simulink model "Ex21"  (R2019b)
settings: Solver=VariableStepAuto  StartTime=0.0  StopTime=10  RelTol=1e-3
values from neighbouring files (symbols this model uses):
  f = 3    [Ex_20.m]    (also in Ex_21.m; Ex_8.m = [0.1 1 1.6 3 16]*1e3; Ex_9.m = 10.^(1 : 0.01 : 5))
  G = 9.8    [Ex_20.m]    (also in Ex_21.m)
  J = 0.4    [Ex_21.m]    (also in Ex_22.m = 1; Ex_23.m = 1.1; Ex_29.m = 1.1; Untitled2.m = 1)
  K = 1    [Ex_10.m]    (also in Ex_21.m; Ex_22.m; Ex_24.m = 1 / qsi^2; Ex_31.m = 4.26)
  M1 = 400    [Ex_20.m]    (also in Ex_21.m = 0.5; Untitled2.m = 1)
  M2 = 20    [Ex_20.m]    (also in Ex_21.m = 1; Untitled2.m = 1)
  R = 0.2    [Ex_21.m]    (also in Ex_22.m; Ex_23.m = 1.3; Ex_27.m = 2*qsi * sqrt(L/C); Ex_29.m = 1.3)
settings Model: Creator=andre  LastModifiedBy=andre

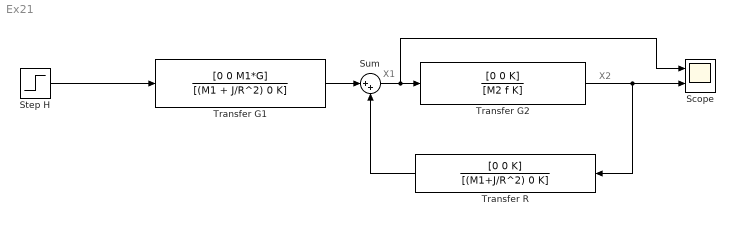
== system Ex21 ==
  note: X1
  note: X2
  Scope : Scope  NumInputPorts=2
  Step H : Step  Time=0  SampleTime=0
  Sum : Sum  Inputs=|++
  Transfer G1 : TransferFcn  Numerator=[0 0 M1*G]  Denominator=[(M1 + J/R^2) 0 K]
  Transfer G2 : TransferFcn  Numerator=[0 0 K]  Denominator=[M2 f K]
  Transfer R : TransferFcn  Numerator=[0 0 K]  Denominator=[(M1+J/R^2) 0 K]
  wires:
  Transfer G2/1 -> Transfer R/1, Scope/2
  Step H/1 -> Transfer G1/1
  Transfer G1/1 -> Sum/1
  Transfer R/1 -> Sum/2
  Sum/1 -> Scope/1, Transfer G2/1
